simulink subsystem "burst_detector"  (R2020a)
settings: Solver=VariableStepAuto  StartTime=0.0  StopTime=10.0  RelTol=1e-3
settings Model: Creator=Philip  LastModifiedBy=Philip

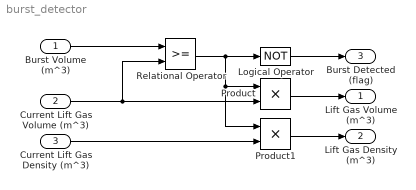
== system burst_detector ==
  Burst Volume (m^3) : Inport
  Current Lift Gas Volume (m^3) : Inport  Port=2
  Current Lift Gas Density (m^3) : Inport  Port=3
  Logical Operator : Logic  Operator=NOT  AllPortsSameDT=off  OutDataTypeStr=boolean
  Product : Product
  Product1 : Product
  Relational Operator : RelationalOperator  OutDataTypeStr=boolean  RndMeth=Simplest
  Lift Gas Volume (m^3) : Outport
  Lift Gas Density (m^3) : Outport  Port=2
  Burst Detected (flag) : Outport  Port=3
  wires:
  Product1/1 -> Lift Gas Density (m^3)/1
  Product/1 -> Lift Gas Volume (m^3)/1
  Current Lift Gas Density (m^3)/1 -> Product1/2
  Relational Operator/1 -> Product/1, Product1/1, Logical Operator/1
  Current Lift Gas Volume (m^3)/1 -> Relational Operator/2, Product/2
  Burst Volume (m^3)/1 -> Relational Operator/1
  Logical Operator/1 -> Burst Detected (flag)/1
